simulink model "simu_Travail1"  (R2016a)
settings: Solver=VariableStepAuto  StartTime=0.0  StopTime=10  RelTol=1e-3
undefined symbols (not defined in the file or in its folder): a, b, Lambdaf
settings Model: Creator=e1401454  LastModifiedBy=e1401454

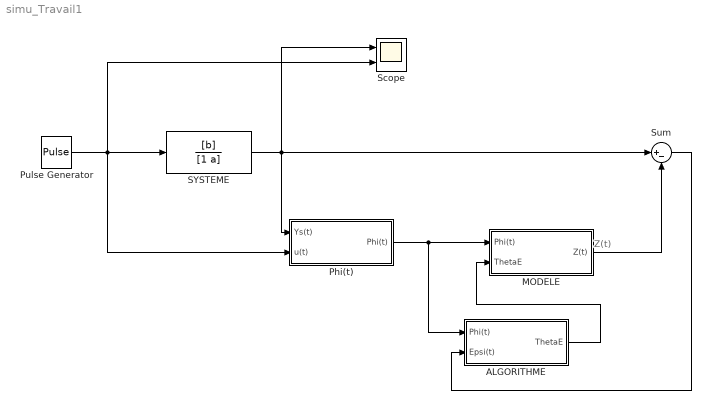
== system simu_Travail1 ==
  note: Z(t)
  "ALGORITHME " : Subsystem
  MODELE : Subsystem
  Phi(t) : Subsystem
  Pulse Generator : DiscretePulseGenerator  PulseType=Time based  Period=1  PulseWidth=50
  SYSTEME : TransferFcn  Numerator=[b]  Denominator=[1 a]
  Scope : Scope  NumInputPorts=2
  Sum : Sum  Inputs=|+-
  wires:
  SYSTEME/1 -> Scope/1, Phi(t)/1(Ys(t)), Sum/1
  Phi(t)/1("Phi(t) ") -> "ALGORITHME "/1(Phi(t)), MODELE/1(Phi(t))
  MODELE/1(Z(t)) -> Sum/2
  "ALGORITHME "/1(ThetaE) -> MODELE/2(ThetaE)
  Sum/1 -> "ALGORITHME "/2("Epsi(t) ")
  Pulse Generator/1 -> Scope/2, Phi(t)/2(u(t)), SYSTEME/1

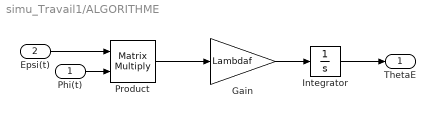
== system simu_Travail1/ALGORITHME  ==
  Phi(t) : Inport
  "Epsi(t) " : Inport  Port=2
  Gain : Gain  Gain=Lambdaf
  Integrator : Integrator
  Product : Product  Multiplication=Matrix(*)
  ThetaE : Outport
  wires:
  "Epsi(t) "/1 -> Product/1
  Phi(t)/1 -> Product/2
  Integrator/1 -> ThetaE/1
  Product/1 -> Gain/1
  Gain/1 -> Integrator/1

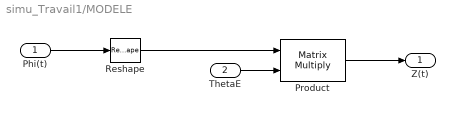
== system simu_Travail1/MODELE ==
  Phi(t) : Inport
  ThetaE : Inport  Port=2
  Product : Product  Multiplication=Matrix(*)
  Reshape : Reshape  OutputDimensionality=Customize  OutputDimensions=[2,1]
  Z(t) : Outport
  wires:
  ThetaE/1 -> Product/2
  Product/1 -> Z(t)/1
  Phi(t)/1 -> Reshape/1
  Reshape/1 -> Product/1

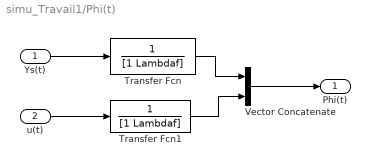
== system simu_Travail1/Phi(t) ==
  Ys(t) : Inport
  u(t) : Inport  Port=2
  Transfer Fcn : TransferFcn  Denominator=[1 Lambdaf]
  Transfer Fcn1 : TransferFcn  Denominator=[1 Lambdaf]
  Vector Concatenate : Concatenate
  "Phi(t) " : Outport
  wires:
  Ys(t)/1 -> Transfer Fcn/1
  u(t)/1 -> Transfer Fcn1/1
  Transfer Fcn/1 -> Vector Concatenate/1
  Transfer Fcn1/1 -> Vector Concatenate/2
  Vector Concatenate/1 -> "Phi(t) "/1
